simulink model "shem_1"  (R2018b)
settings: Solver=VariableStepAuto  StartTime=0.0  StopTime=600  RelTol=1e-3
settings Model: Creator=murad  LastModifiedBy=murad

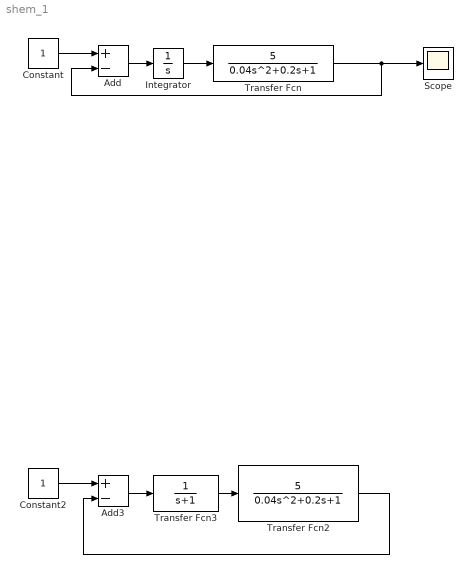
== system shem_1 ==
  Add : Sum  Inputs=+-
  Add3 : Sum  Inputs=+-
  Constant : Constant
  Constant2 : Constant
  Integrator : Integrator
  Scope : Scope
  Transfer Fcn : TransferFcn  Numerator=[5]  Denominator=[0.04 0.2 1]
  Transfer Fcn2 : TransferFcn  Numerator=[5]  Denominator=[0.04 0.2 1]
  Transfer Fcn3 : TransferFcn  Denominator=[1 1]
  wires:
  Constant/1 -> Add/1
  Add/1 -> Integrator/1
  Constant2/1 -> Add3/1
  Transfer Fcn2/1 -> Add3/2
  Add3/1 -> Transfer Fcn3/1
  Transfer Fcn3/1 -> Transfer Fcn2/1
  Integrator/1 -> Transfer Fcn/1
  Transfer Fcn/1 -> Add/2, Scope/1
